simulink model "modelo_pid"  (R2018a)
settings: Solver=FixedStepAuto  StartTime=0.0  StopTime=0.1  FixedStep=0.0001  RelTol=1e-3
values from neighbouring files (symbols this model uses):
  A = [0 0 1 0;0 0 0 1;k 0 0 x;0 k -x 0]    [autovalores.m]    (also in graficoim.m = 0.0004; sim1.m = [zeros(2) eye(2);Ke*eye(2) -Ge]; sim2.m = [zeros(2) eye(2);Ke*eye(2) -Ge])
  B = kb*[zeros(2);eye(2)]    [autovalores.m]    (also in sim1.m = (1/J)*d*b*ki*[zeros(2);eye(2)]; sim2.m = (1/J)*d*b*ki*[zeros(2);eye(2)])
  C = [eye(2) zeros(2)]    [autovalores.m]    (also in sim1.m; sim2.m)
  F = Fdn    [sim1.m]    (also in sim2.m)
  omega = 4000    [sim1.m]    (also in sim2.m)
  x0 = [0.0002;-0.0002;0;0]    [sim1.m]    (also in sim2.m)
undefined symbols (not defined in the file or in its folder): L
settings Model: Creator=vinic  LastModifiedBy=vinic

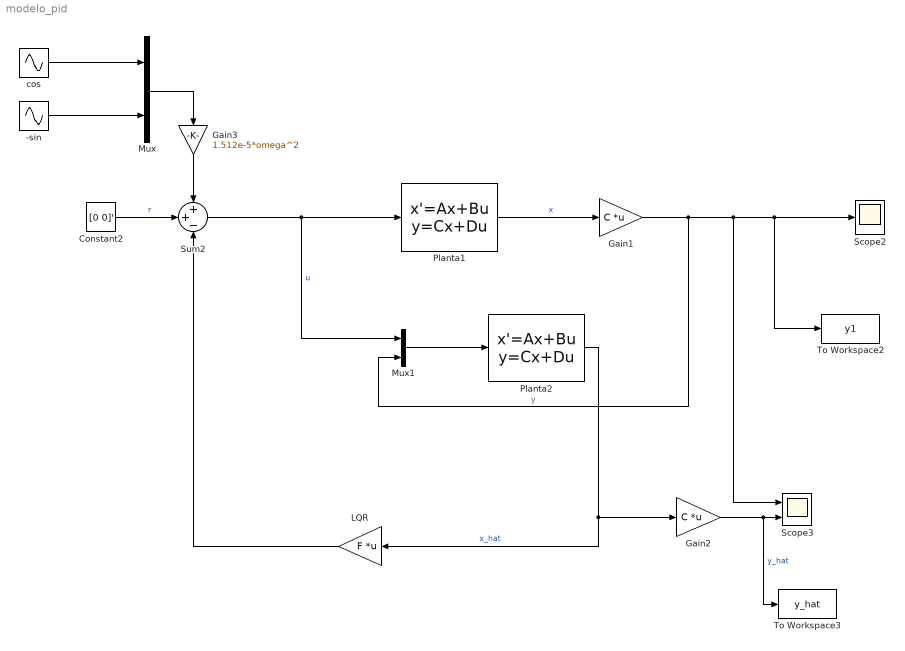
== system modelo_pid ==
  -sin : Sin  Amplitude=1.512e-6*omega^2  Frequency=omega  SampleTime=0
  Constant2 : Constant  Value=[0 0]'
  Gain1 : Gain  Gain=C  Multiplication=Matrix(K*u)
  Gain2 : Gain  Gain=C  Multiplication=Matrix(K*u)
  Gain3 : Gain  Gain=1.512e-5*omega^2
  LQR : Gain  Gain=F  Multiplication=Matrix(K*u)
  Mux : Mux  Inputs=2
  Mux1 : Mux  Inputs=2
  Planta1 : StateSpace  A=A  B=B  C=eye(4)  D=zeros(4,2)  InitialCondition=x0
  Planta2 : StateSpace  A=A-L*C  B=[B L]  C=eye(4)  D=zeros(4,4)  InitialCondition=[0;0;0;0]
  Scope2 : Scope
  Scope3 : Scope  NumInputPorts=2
  Sum2 : Sum  Inputs=++-
  To Workspace2 : ToWorkspace  VariableName=y1  SampleTime=-1
      settings: Save2DSignal=2-D array (concatenate along first dimension)
  To Workspace3 : ToWorkspace  VariableName=y_hat  SampleTime=-1
      settings: Save2DSignal=2-D array (concatenate along first dimension)
  cos : Sin  Amplitude=1.512e-6*omega^2  Frequency=omega  SampleTime=0
  wires:
  Mux1/1 -> Planta2/1
  Planta2/1 -> Gain2/1, LQR/1  "x_hat"
  Gain2/1 -> To Workspace3/1, Scope3/2  "y_hat"
  Gain1/1 -> Scope3/1, To Workspace2/1, Scope2/1, Mux1/2  "y"
  Planta1/1 -> Gain1/1  "x"
  Sum2/1 -> Planta1/1, Mux1/1  "u"
  cos/1 -> Mux/1
  -sin/1 -> Mux/2
  Constant2/1 -> Sum2/2  "r"
  LQR/1 -> Sum2/3
  Gain3/1 -> Sum2/1
  Mux/1 -> Gain3/1
